simulink model "DCMotorModel_Sim"  (R2021a)
settings: Solver=ode45  StartTime=0.0  StopTime=2  RelTol=1e-3  EnableMultiTasking=on
values from neighbouring files (symbols this model uses):
  b = 3.5077E-6    (= 3.5077e-06)    [DCMotorModel_Run.m]
  J = 3.2284E-6    (= 3.2284e-06)    [DCMotorModel_Run.m]
  Kb = 0.0274    [DCMotorModel_Run.m]
  Kt = 0.0274    [DCMotorModel_Run.m]
  L = 2.75E-6    (= 2.75e-06)    [DCMotorModel_Run.m]
  R = 4    [DCMotorModel_Run.m]
  V = 1    [DCMotorModel_Run.m]
settings Model: Creator=DZR3QN  LastModifiedBy=moham
settings SolverCC: AlgebraicLoopSolver=TrustRegion
settings DataIOCC: LimitDataPoints=on  SaveFormat=Array  ReturnWorkspaceOutputs=off
settings OptimizationCC: LifeSpan=inf
settings DebuggingCC: SolverPrmCheckMsg=warning  SFUnexpectedBacktrackingDiag=warning  SFNoUnconditionalDefaultTransitionDiag=warning  SFExecutionAtInitializationDiag=none  SFMachineParentedDataDiag=warning  ArithmeticOperatorsInVariantConditions=warning
settings HardwareCC: ProdBitPerPointer=32  ProdBitPerSizeT=32  ProdBitPerPtrDiffT=32  ProdLargestAtomicFloat=None  ProdIntDivRoundTo=Undefined  ProdEndianess=Unspecified  ProdWordSize=32  ProdHWDeviceType=32-bit Generic
settings ModelReferenceCC: PropagateSignalLabelsOutOfModel=off
settings SFSimCC: SimUseLocalCustomCode=off  CustomCodeUndefinedFunction=UseInterfaceOnly
settings RTWCC: RTWUseLocalCustomCode=off
settings CodeAppCC: StateflowObjectComments=on
settings GRTTargetCC: TargetLangStandard=C89/C90 (ANSI)
settings ConfigComp: CovMetricSettings=dw  CovSaveCumulativeToWorkspaceVar=on  CovSaveSingleToWorkspaceVar=on  CovExternalEMLEnable=off  CovSFcnEnable=off

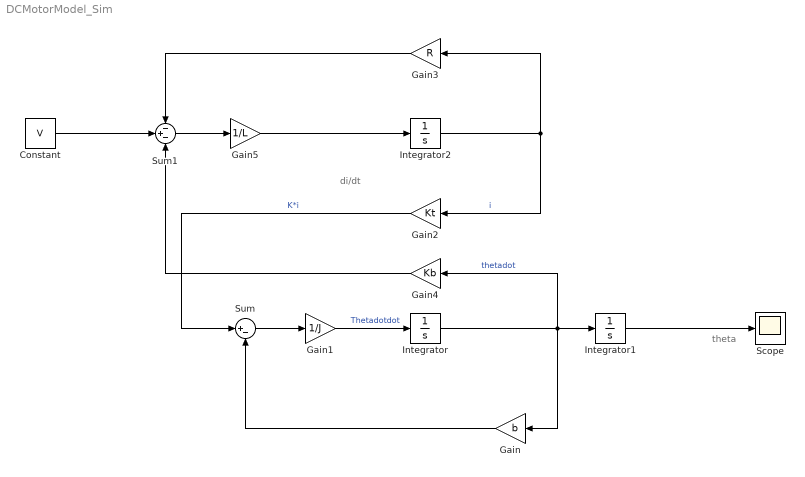
== system DCMotorModel_Sim ==
  note: di/dt
  note: theta
  Constant : Constant  Value=V
  Gain : Gain  Gain=b
  Gain1 : Gain  Gain=1/J
  Gain2 : Gain  Gain=Kt
  Gain3 : Gain  Gain=R
  Gain4 : Gain  Gain=Kb
  Gain5 : Gain  Gain=1/L
  Integrator : Integrator
  Integrator1 : Integrator
  Integrator2 : Integrator
  Scope : Scope
  Sum : Sum  Inputs=|+-
  Sum1 : Sum  Inputs=-+-
  wires:
  Gain1/1 -> Integrator/1  "Thetadotdot"
  Integrator/1 -> Gain4/1, Gain/1, Integrator1/1  "thetadot"
  Integrator1/1 -> Scope/1
  Gain/1 -> Sum/2
  Gain2/1 -> Sum/1  "K*i"
  Sum/1 -> Gain1/1
  Gain5/1 -> Integrator2/1
  Integrator2/1 -> Gain2/1, Gain3/1  "i"
  Gain3/1 -> Sum1/1
  Constant/1 -> Sum1/2
  Gain4/1 -> Sum1/3
  Sum1/1 -> Gain5/1
